simulink model "z_noise"  (R2014a)
settings: Solver=ode45  StartTime=0.0  StopTime=2000  RelTol=1e-3
values from neighbouring files (symbols this model uses):
  Sample_Time = 1    [main.m]
libraries: dspsrcs4 x1
settings Model: Creator=User  LastModifiedBy=User

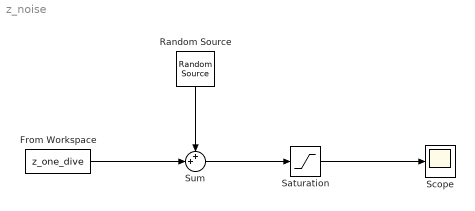
== system z_noise ==
  From Workspace : FromWorkspace  VariableName=z_one_dive  SampleTime=Sample_Time  Interpolate=off  OutputAfterFinalValue=Cyclic repetition
  Random Source : dspsrcs4/Random Source  SrcType=Gaussian  NormMethod=Ziggurat  CltLength=12  MinVal=0  MaxVal=1  MeanVal=.01  VarVal=.022  RepMode=Not repeatable  rawSeed=1  IsInherit=on  SampMode=Continuous  SampTime=1  SampFrame=1  DataType=Single  OutComplex=Real
  Saturation : Saturate  UpperLimit=1  LowerLimit=0
  Scope : Scope
  Sum : Sum  Inputs=++|
  wires:
  Sum/1 -> Saturation/1
  From Workspace/1 -> Sum/2
  Random Source/1 -> Sum/1
  Saturation/1 -> Scope/1
